simulink library "Audiopilot_3_5"  (R2022b)
settings: Solver=VariableStepAuto  StartTime=0.0  StopTime=10.0  RelTol=1e-3
values from neighbouring files (symbols this model uses):
  NumHFRefLPF = 4    [Audiopilot_3_5Mask.m]
  NumLFRef = 1    [Audiopilot_3_5Mask.m]
  NumMicChannels = 1    [Audiopilot_3_5Mask.m]
  NumMusicChannels = 6    [Audiopilot_3_5Mask.m]
undefined symbols (not defined in the file or in its folder): Row
libraries: TuneVar x11, StateVar x5, HandyTextFile x4, RTC x4, TOP x4, FeaturePath x3, Compensation x2, HighFrequencyNoiseEstimatorCoh x2, SpeedBoundsNoiseSlew x2, LowFrequencyNoiseEstimatorCoh x1
settings Model: Creator=sc10652  LastModifiedBy=db1045444
settings SolverCC: AlgebraicLoopSolver=TrustRegion
settings DataIOCC: ReturnWorkspaceOutputs=off
settings DebuggingCC: UnconnectedInputMsg=warning  UnconnectedOutputMsg=warning  UnconnectedLineMsg=warning  SFMachineParentedDataDiag=warning  ArithmeticOperatorsInVariantConditions=warning
settings ModelReferenceCC: EnableRefExpFcnMdlSchedulingChecks=on
settings SFSimCC: CustomCodeUndefinedFunction=UseInterfaceOnly

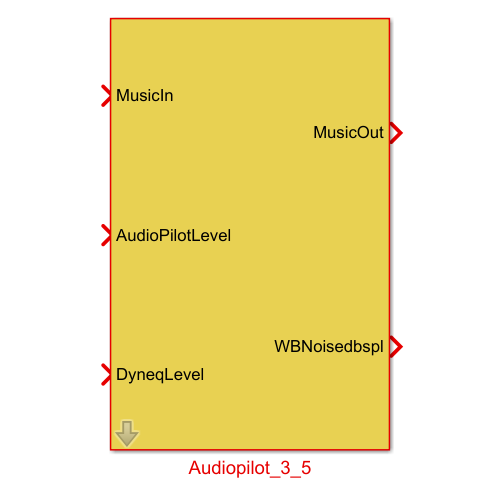
[thumbnail: Simulink's stored preview of the top-level diagram]
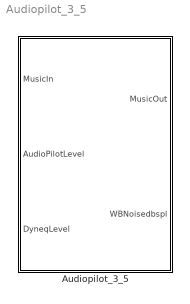
== system Audiopilot_3_5 ==
  Audiopilot_3_5 : Subsystem  mask(AudioPilot 3.5){FeatureName=Audiopilot, InputAudioMode=Stereo - 2 Channels, NoiseEstimationMode=Speed Only, IncludeSpumTails=on, IncludeIgnoreMicFlag=on, Config=[]}
      mask prompts: FeatureName "Feature Name:"; InputAudioMode "Input Audio Mode"; NoiseEstimationMode "Mode"; IncludeSpumTails "Include SPUM Tails as Reference Channels for High-Frequency Noise Estimator"; IncludeIgnoreMicFlag "Include Ignore Microphone Flag as Input"; Config "Audiopilot_3_5Config"
      mask help:
      | This is the top level model implementing AudioPilot 3.5.
      | It is configurable to accommodate both stereo inputs and surround inputs.  It can also reconfigure itself to become a speed-only implementation. For the regular implementation, there are two options. One is to allow a flag signal to instruct the algorithm to ignore the microphone signal; the other is to include in the set of "high-passed" reference channels the 2 channels representing the SPUM tails from the Medusa Upmixer.
      | Build Time Configuration settings typically set for this block include the frame size and the sample rate of the input audio. Other options include the type of code generation and whether all RTC blocks will generate a response.
      mask init:
      | blkh = gcbh;
      | 
      | Config = BTConfig.Assert(blkh,Config);
      | Config.Validate();
      | 
      | FrameSize = Config.FrameSize;
      | SampleRate = Config.SampleRateHz;
      |  
      | % Make the choice for the Noise Estimation Variant
      | Audiopilot_3_5Mask.ConfigureVariant(blkh,NoiseEstimationMode);
      | 
      | % Set up the number of audio channels for each input
      | [NumMicChannels,NumMusicChannels, ...
      |     NumHFRefLPF,NumHFRefBPF,NumLFRef] = ...
      |     Audiopilot_3_5Mask.ChannelSetUp(blkh,InputAudioMode,...
      |                 NoiseEstimationMode,IncludeSpumTails);
      | 
      | % Configure RTC responses            
      | Audiopilot_3_5Mask.ConfigureRtcResponses(blkh,...
      |                 Config.EnableRtcResponse)           
      | 
      | % Configure the Model according to Mask Parameters   
      | Audiopilot_3_5Mask.ConfigureModel(blkh,InputAudioMode,...
      |     NoiseEstimationMode,IncludeIgnoreMicFlag);
      | 
      | BTConfig.InitSetFeatureIfPresent(blkh,'FeatureName');
      mask TypeOptions FeatureName: FeaturePath/FeatureName
      mask TypeOptions InputAudioMode: Stereo - 2 Channels | Surround - 6 Channels
      mask TypeOptions NoiseEstimationMode: Regular | Speed Only
      mask Callback NoiseEstimationMode: Audiopilot_3_5Mask.NoiseEstimationModeCallBack(gcbh);
      mask Callback Config: BTConfig.CallbackHideIfPresent(gcbh,{'FeatureName'});
      mask DialogControl DTCTitle Prompt: <b> Design Time Configuration </b>
      mask DialogControl NoiseEstimationBox Prompt: Noise Estimation
      mask DialogControl BTCTitle Prompt: <b> Build Time Configuration </b>

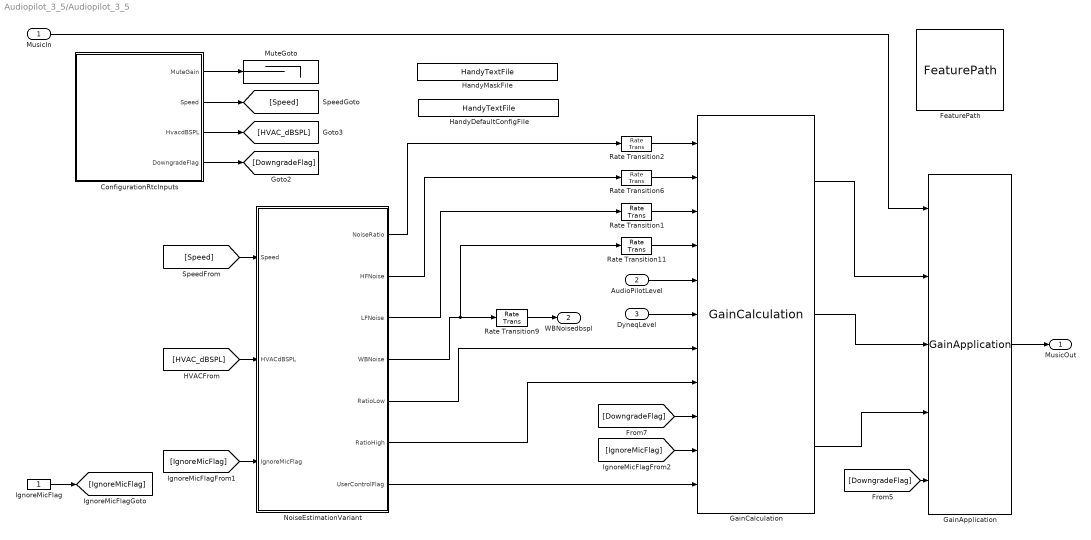
== system Audiopilot_3_5/Audiopilot_3_5 ==
  MusicIn : Inport  OutDataTypeStr=single  PortDimensions=[FrameSize NumMusicChannels]
  AudioPilotLevel : Inport  Port=2  OutDataTypeStr=single  PortDimensions=1
  DyneqLevel : Inport  Port=3  OutDataTypeStr=single  PortDimensions=1
  ConfigurationRtcInputs : Subsystem
  FeaturePath : FeaturePath/FeaturePath  FeatureName=Audiopilot  IsGroup=off  GroupNumber=-1  IsModule=off  TriggerInit=[1175 264 1290 371]
      settings: SourceProductName=Bose Talaria
  GainApplication : Compensation/GainApplication  NumInputChannels=NumMusicChannels  Config=Config.GainApp
  GainCalculation : Compensation/GainCalculation  Config=Config.GainCalc
  HandyDefaultConfigFile : HandyTextFile/HandyTextFile  TemplateSource=Config  FileSuffix=Init  OpenDialogOnLoad=off  UseThisBlockName=off  TheDefaultText=|  ShowInLibBrowser=on
      | % $(FILENAME) Setup model parameters for each "Init" callback (e.g. update diagram)
      | sample_rate_in_hertz = 44100;
      | frame_size = 32;
      | sysin_channel_count = 2;
      settings: SourceProductName=Bose Talaria
  HandyMaskFile : HandyTextFile/HandyTextFile  TemplateSource=Mask  FileSuffix=Init  OpenDialogOnLoad=off  UseThisBlockName=off  TheDefaultText=|  ShowInLibBrowser=on
      | % $(FILENAME) Setup model parameters for each "Init" callback (e.g. update diagram)
      | sample_rate_in_hertz = 44100;
      | frame_size = 32;
      | sysin_channel_count = 2;
      settings: SourceProductName=Bose Talaria
  IgnoreMicFlag : Constant  OutDataTypeStr=boolean
  MuteGoto : Terminator
  NoiseEstimationVariant : Subsystem  Variant=on  VariantControlMode=label  LabelModeActiveChoice=Speed Only  PropagateVariantConditions=on
  Rate Transition{1..2,6,9,11} (5 alike) : RateTransition  Deterministic=off
  MusicOut : Outport  VectorParamsAs1DForOutWhenUnconnected=off
  WBNoisedbspl : Outport  Port=2  VectorParamsAs1DForOutWhenUnconnected=off
  wires:
  [HVAC_dBSPL] -> NoiseEstimationVariant/2(HVACdBSPL)
  [Speed] -> NoiseEstimationVariant/1(Speed)
  NoiseEstimationVariant/3(LFNoise) -> Rate Transition1/1
  NoiseEstimationVariant/2(HFNoise) -> Rate Transition6/1
  NoiseEstimationVariant/1(NoiseRatio) -> Rate Transition2/1
  ConfigurationRtcInputs/1(MuteGain) -> MuteGoto/1
  ConfigurationRtcInputs/3(HvacdBSPL) -> [HVAC_dBSPL]
  ConfigurationRtcInputs/2(Speed) -> [Speed]
  ConfigurationRtcInputs/4(DowngradeFlag) -> [DowngradeFlag]
  [DowngradeFlag] -> GainCalculation/9
  GainCalculation/2 -> GainApplication/3
  NoiseEstimationVariant/4(WBNoise) -> Rate Transition11/1, Rate Transition9/1
  Rate Transition6/1 -> GainCalculation/2
  MusicIn/1 -> GainApplication/1
  NoiseEstimationVariant/7("UserControlFlag ") -> GainCalculation/11
  Rate Transition1/1 -> GainCalculation/3
  Rate Transition11/1 -> GainCalculation/4
  GainCalculation/1 -> GainApplication/2
  [DowngradeFlag] -> GainApplication/5
  DyneqLevel/1 -> GainCalculation/6
  Rate Transition2/1 -> GainCalculation/1
  AudioPilotLevel/1 -> GainCalculation/5
  GainApplication/1 -> MusicOut/1
  GainCalculation/3 -> GainApplication/4
  Rate Transition9/1 -> WBNoisedbspl/1
  NoiseEstimationVariant/5(RatioLow) -> GainCalculation/7
  NoiseEstimationVariant/6(RatioHigh) -> GainCalculation/8
  [IgnoreMicFlag] -> GainCalculation/10
  IgnoreMicFlag/1 -> [IgnoreMicFlag]
  [IgnoreMicFlag] -> NoiseEstimationVariant/3(IgnoreMicFlag)

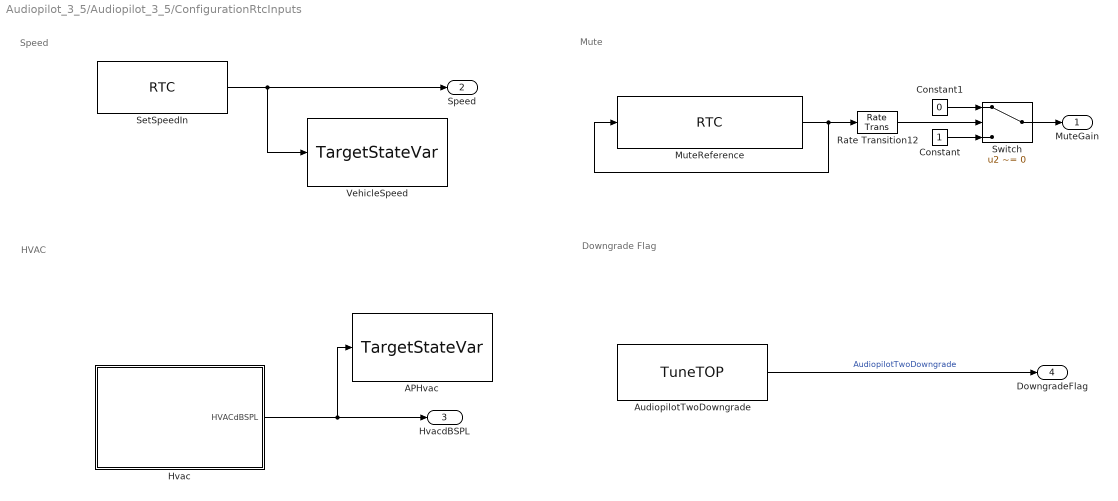
== system Audiopilot_3_5/Audiopilot_3_5/ConfigurationRtcInputs ==
  note: Mute
  note: Speed
  note: HVAC
  note: Downgrade Flag
  APHvac : StateVar/TargetStateVar  TriggerInit=[1390 1281 1530 1349]  TspName=HvacDbspl  StateName=HvacDbspl  UseSameName=on  IfdefMacro=[]
      settings: SourceProductName=Bose Talaria
  AudiopilotTwoDowngrade : TuneVar/TuneTOP  TriggerInit=[1655 1312 1805 1368]  TopName=TwoDowngrade  TuneName=TwoDowngrade  DataType=uint32  TunabilityNumber=1  MinValue=[]  MaxValue=[]  BankNumber=0  PreOverlay=false  PostOverlay=false  UseSameName=on  MaskValue=0
      settings: SourceProductName=Bose Talaria
  Constant : Constant  OutDataTypeStr=single
  Constant1 : Constant  Value=0  OutDataTypeStr=single
  Hvac : Subsystem  mask(AudioPilot - HVAC Table){Config=Config.HVAC}
      mask prompts: Config "HVACConfig"
      mask help: This block implements the table lookup for the HVAC index. It has 16 entries and returns the HVAC level in dBSPL.
      mask init:
      | blkh = gcbh;
      | 
      | Config = BTConfig.Assert(blkh,Config);
      | Config.Validate();
      | 
      | MaskHvacTableSize = Config.HVACTableSize;
      mask Help:
      | This block implements the table lookup for the HVAC index.  It has 16 entries and returns the HVAC level in dBSPL.
      | 
      | Arguments for this block:
      | 
      | Configuration
      | The block can be configured using an object of class, HVACConfig.  If the "use Default Configuration Only" box is checked, then this option is disabled.
      mask DialogControl BTC Prompt: Build Time Configuration
      mask DialogControl Config Tooltip: The configuration has to be an object of the class, HVACConfig.
  MuteReference : RTC/RTC  REQ_Priority=RTC_Mask.NormalPriority  RequestAtInit=off  EnableRequest=off  REQElemName1=muteReference  REQElemType1=uint32  REQElemWidth1=1  REQElemInitial1=0  REQElemType2=uint32  REQElemWidth2=1  REQElemInitial2=[]  REQElemType3=uint32  REQElemWidth3=1  REQElemInitial3=[]  REQElemType4=uint32  REQElemWidth4=1  REQElemInitial4=[]  REQElemType5=uint32  REQElemWidth5=1  REQElemInitial5=[]  REQElemType6=uint32  REQElemWidth6=1  REQElemInitial6=[]  REQElemType7=uint32  REQElemWidth7=1  REQElemInitial7=[]  REQElemType8=uint32  REQElemWidth8=1  REQElemInitial8=[]  REQElemType9=uint32  REQElemWidth9=1  REQElemInitial9=[]  REQElemType10=uint32  REQElemWidth10=1  REQElemInitial10=[]  EnableResponse=on  EnableRSP_StatusIn=off  RSPElemName1=muteReference  RSPElemType1=uint32  RSPElemWidth1=1  RSPElemType2=uint32  RSPElemWidth2=1  RSPElemType3=uint32  RSPElemWidth3=1  RSPElemType4=uint32  RSPElemWidth4=1  RSPElemType5=uint32  RSPElemWidth5=1  RSPElemType6=uint32  RSPElemWidth6=1  RSPElemType7=uint32  RSPElemWidth7=1  RSPElemType8=uint32  RSPElemWidth8=1  RSPElemType9=uint32  RSPElemWidth9=1  RSPElemType10=uint32  RSPElemWidth10=1  EnableNotification=off  EnableNTF_PrepTrig=off  NTFElemName1=freezeAdapt  NTFElemType1=single  NTFElemWidth1=1  NTFElemType2=uint32  NTFElemWidth2=1  NTFElemType3=uint32  NTFElemWidth3=1  NTFElemType4=uint32  NTFElemWidth4=1  NTFElemType5=uint32  NTFElemWidth5=1  NTFElemType6=uint32  NTFElemWidth6=1  NTFElemType7=uint32  NTFElemWidth7=1  NTFElemType8=uint32  NTFElemWidth8=1  NTFElemType9=uint32  NTFElemWidth9=1  NTFElemType10=uint32  NTFElemWidth10=1  MaskMessageName=muteReference
      settings: SourceProductName=Bose Talaria
  Rate Transition12 : RateTransition  Deterministic=off
  SetSpeedIn : RTC/RTC  REQ_Priority=RTC_Mask.NormalPriority  RequestAtInit=off  EnableRequest=off  REQElemName1=speedIn  REQElemType1=single  REQElemWidth1=1  REQElemInitial1=[]  REQElemType2=single  REQElemWidth2=1  REQElemInitial2=[]  REQElemType3=uint32  REQElemWidth3=1  REQElemInitial3=[]  REQElemType4=uint32  REQElemWidth4=1  REQElemInitial4=[]  REQElemType5=uint32  REQElemWidth5=1  REQElemInitial5=[]  REQElemType6=uint32  REQElemWidth6=1  REQElemInitial6=[]  REQElemType7=uint32  REQElemWidth7=1  REQElemInitial7=[]  REQElemType8=uint32  REQElemWidth8=1  REQElemInitial8=[]  REQElemType9=uint32  REQElemWidth9=1  REQElemInitial9=[]  REQElemType10=uint32  REQElemWidth10=1  REQElemInitial10=[]  EnableResponse=off  EnableRSP_StatusIn=off  RSPElemType1=single  RSPElemWidth1=1  RSPElemType2=uint32  RSPElemWidth2=1  RSPElemType3=uint32  RSPElemWidth3=1  RSPElemType4=uint32  RSPElemWidth4=1  RSPElemType5=uint32  RSPElemWidth5=1  RSPElemType6=uint32  RSPElemWidth6=1  RSPElemType7=uint32  RSPElemWidth7=1  RSPElemType8=uint32  RSPElemWidth8=1  RSPElemType9=uint32  RSPElemWidth9=1  RSPElemType10=uint32  RSPElemWidth10=1  EnableNotification=off  EnableNTF_PrepTrig=off  NTFElemType1=uint32  NTFElemWidth1=1  NTFElemType2=uint32  NTFElemWidth2=1  NTFElemType3=uint32  NTFElemWidth3=1  NTFElemType4=uint32  NTFElemWidth4=1  NTFElemType5=uint32  NTFElemWidth5=1  NTFElemType6=uint32  NTFElemWidth6=1  NTFElemType7=uint32  NTFElemWidth7=1  NTFElemType8=uint32  NTFElemWidth8=1  NTFElemType9=uint32  NTFElemWidth9=1  NTFElemType10=uint32  NTFElemWidth10=1  MaskMessageName=setSpeedIn
      settings: SourceProductName=Bose Talaria
  Switch : Switch  Criteria=u2 ~= 0  OutDataTypeStr=single  SaturateOnIntegerOverflow=off  InputSameDT=off
  VehicleSpeed : StateVar/TargetStateVar  TriggerInit=[1345 1086 1485 1154]  TspName=VehicleSpeed  StateName=VehicleSpeed  UseSameName=on  IfdefMacro=[]
      settings: SourceProductName=Bose Talaria
  MuteGain : Outport  OutDataTypeStr=single  VectorParamsAs1DForOutWhenUnconnected=off
  Speed : Outport  Port=2  VectorParamsAs1DForOutWhenUnconnected=off
  HvacdBSPL : Outport  Port=3  VectorParamsAs1DForOutWhenUnconnected=off
  DowngradeFlag : Outport  Port=4  VectorParamsAs1DForOutWhenUnconnected=off
  wires:
  MuteReference/1 -> Rate Transition12/1, MuteReference/1
  Rate Transition12/1 -> Switch/2
  SetSpeedIn/1 -> VehicleSpeed/1, Speed/1
  AudiopilotTwoDowngrade/1 -> DowngradeFlag/1  "AudiopilotTwoDowngrade"
  Hvac/1(HVACdBSPL) -> APHvac/1, HvacdBSPL/1
  Constant/1 -> Switch/3
  Switch/1 -> MuteGain/1
  Constant1/1 -> Switch/1

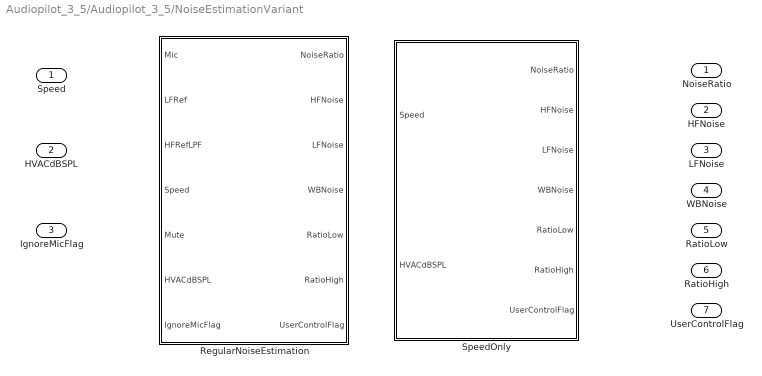
== system Audiopilot_3_5/Audiopilot_3_5/NoiseEstimationVariant ==
  Speed : Inport
  HVACdBSPL : Inport  Port=2
  IgnoreMicFlag : Inport  Port=3
  RegularNoiseEstimation : Subsystem  VariantControl=Regular
  SpeedOnly : Subsystem  VariantControl=Speed Only  mask(AudioPilot - Speed Only Noise Estimation){Config=Config.SpeedOnly}
      mask prompts: Config "SpeedOnlyConfig"
      mask help: This block implements the speed only variant for noise estimation
      mask init:
      | blkh = gcbh;
      | 
      | Config = BTConfig.Assert(blkh,Config);
      | Config.Validate();
      | 
      | SampleRate = Config.SampleRateHz;
      | DecRate = Config.DecRateHz;
      mask Help:
      | This block implements the speed only variant for noise estimation.
      | 
      | Arguments for this block:
      | 
      | Configuration
      | The block can be configured using an object of class, SpeedOnlyConfig.  If the "use Default Configuration Only" box is checked, then this option is disabled.
      | 
      | Sample Rate
      | This is the sample rate of the input audio streams, typically 44100 Hz or 48 kHz.
      mask DialogControl BTC Prompt: Build Time Configuration
      mask DialogControl Config Tooltip: The configuration has to be an object of the class, SpeedOnlyConfig.
  NoiseRatio : Outport  VectorParamsAs1DForOutWhenUnconnected=off
  HFNoise : Outport  Port=2  VectorParamsAs1DForOutWhenUnconnected=off
  LFNoise : Outport  Port=3  VectorParamsAs1DForOutWhenUnconnected=off
  WBNoise : Outport  Port=4  VectorParamsAs1DForOutWhenUnconnected=off
  RatioLow : Outport  Port=5  VectorParamsAs1DForOutWhenUnconnected=off
  RatioHigh : Outport  Port=6  VectorParamsAs1DForOutWhenUnconnected=off
  "UserControlFlag " : Outport  Port=7  VectorParamsAs1DForOutWhenUnconnected=off

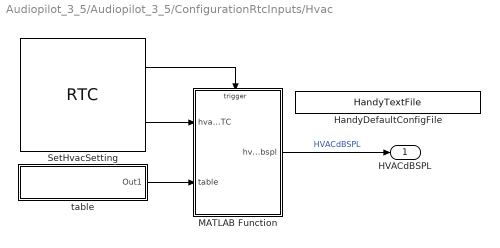
== system Audiopilot_3_5/Audiopilot_3_5/ConfigurationRtcInputs/Hvac ==
  HandyDefaultConfigFile : HandyTextFile/HandyTextFile  TemplateSource=Config  FileSuffix=Init  OpenDialogOnLoad=off  UseThisBlockName=off  TheDefaultText=|  ShowInLibBrowser=on
      | % $(FILENAME) Setup model parameters for each "Init" callback (e.g. update diagram)
      | sample_rate_in_hertz = 44100;
      | frame_size = 32;
      | sysin_channel_count = 2;
      settings: SourceProductName=Bose Talaria
  MATLAB Function : MATLAB Function  TreatAsAtomicUnit=on
  SetHvacSetting : RTC/RTC  REQ_Priority=RTC_Mask.NormalPriority  RequestAtInit=off  EnableRequest=on  REQElemName1=HVACSetting  REQElemType1=single  REQElemWidth1=1  REQElemInitial1=[]  REQElemType2=single  REQElemWidth2=1  REQElemInitial2=[]  REQElemType3=uint32  REQElemWidth3=1  REQElemInitial3=[]  REQElemType4=uint32  REQElemWidth4=1  REQElemInitial4=[]  REQElemType5=uint32  REQElemWidth5=1  REQElemInitial5=[]  REQElemType6=uint32  REQElemWidth6=1  REQElemInitial6=[]  REQElemType7=uint32  REQElemWidth7=1  REQElemInitial7=[]  REQElemType8=uint32  REQElemWidth8=1  REQElemInitial8=[]  REQElemType9=uint32  REQElemWidth9=1  REQElemInitial9=[]  REQElemType10=uint32  REQElemWidth10=1  REQElemInitial10=[]  EnableResponse=off  EnableRSP_StatusIn=off  RSPElemType1=uint32  RSPElemWidth1=1  RSPElemType2=uint32  RSPElemWidth2=1  RSPElemType3=uint32  RSPElemWidth3=1  RSPElemType4=uint32  RSPElemWidth4=1  RSPElemType5=uint32  RSPElemWidth5=1  RSPElemType6=uint32  RSPElemWidth6=1  RSPElemType7=uint32  RSPElemWidth7=1  RSPElemType8=uint32  RSPElemWidth8=1  RSPElemType9=uint32  RSPElemWidth9=1  RSPElemType10=uint32  RSPElemWidth10=1  EnableNotification=off  EnableNTF_PrepTrig=off  NTFElemType1=uint32  NTFElemWidth1=1  NTFElemType2=uint32  NTFElemWidth2=1  NTFElemType3=uint32  NTFElemWidth3=1  NTFElemType4=uint32  NTFElemWidth4=1  NTFElemType5=uint32  NTFElemWidth5=1  NTFElemType6=uint32  NTFElemWidth6=1  NTFElemType7=uint32  NTFElemWidth7=1  NTFElemType8=uint32  NTFElemWidth8=1  NTFElemType9=uint32  NTFElemWidth9=1  NTFElemType10=uint32  NTFElemWidth10=1  MaskMessageName=setHVACSetting
      settings: SourceProductName=Bose Talaria
  table : Subsystem
  HVACdBSPL : Outport  VectorParamsAs1DForOutWhenUnconnected=off
  wires:
  SetHvacSetting/2 -> MATLAB Function/1(hvacSettingRTC)
  SetHvacSetting/1 -> MATLAB Function/Trigger
  table/1(Out1) -> MATLAB Function/2(table)
  MATLAB Function/1(hvacDbspl) -> HVACdBSPL/1  "HVACdBSPL"

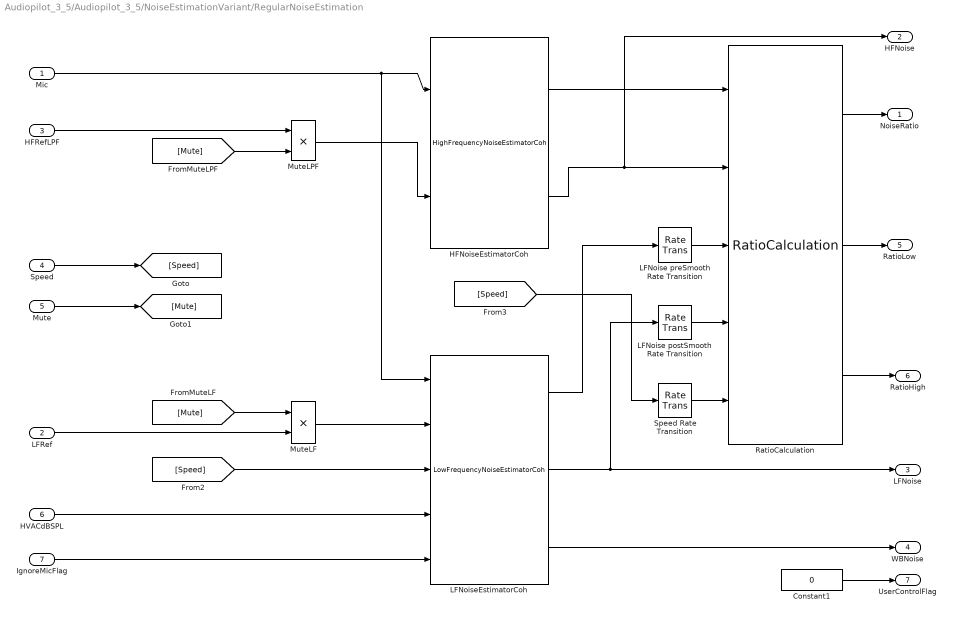
== system Audiopilot_3_5/Audiopilot_3_5/NoiseEstimationVariant/RegularNoiseEstimation ==
  Mic : Inport  PortDimensions=[FrameSize NumMicChannels]
  LFRef : Inport  Port=2  OutDataTypeStr=single  PortDimensions=[FrameSize NumLFRef]
  HFRefLPF : Inport  Port=3  OutDataTypeStr=single  PortDimensions=[FrameSize NumHFRefLPF]
  Speed : Inport  Port=4  OutDataTypeStr=single
  Mute : Inport  Port=5  OutDataTypeStr=single
  HVACdBSPL : Inport  Port=6  OutDataTypeStr=single
  IgnoreMicFlag : Inport  Port=7
  Constant1 : Constant  Value=0  OutDataTypeStr=boolean
  HFNoiseEstimatorCoh : HighFrequencyNoiseEstimatorCoh/HighFrequencyNoiseEstimatorCoh  FeatureName=HfNoise  NumHFRefLPF=NumHFRefLPF  NumHFRefBPF=NumHFRefBPF  Config=Config.HfNoise  TriggerInit=0
  LFNoise postSmooth Rate Transition : RateTransition  Deterministic=off
  LFNoise preSmooth Rate Transition : RateTransition  Deterministic=off
  LFNoiseEstimatorCoh : LowFrequencyNoiseEstimatorCoh/LowFrequencyNoiseEstimatorCoh  FeatureName=LfNoise  Config=Config.LfNoise  TriggerInit=0
  MuteLF : Product  Inputs=**
  MuteLPF : Product  Inputs=**
  RatioCalculation : HighFrequencyNoiseEstimatorCoh/RatioCalculation  FeatureName=Ratio  Config=Config.Ratio
  Speed Rate Transition : RateTransition  Deterministic=off
  NoiseRatio : Outport  VectorParamsAs1DForOutWhenUnconnected=off
  HFNoise : Outport  Port=2  VectorParamsAs1DForOutWhenUnconnected=off
  LFNoise : Outport  Port=3  VectorParamsAs1DForOutWhenUnconnected=off
  WBNoise : Outport  Port=4  VectorParamsAs1DForOutWhenUnconnected=off
  RatioLow : Outport  Port=5  VectorParamsAs1DForOutWhenUnconnected=off
  RatioHigh : Outport  Port=6  VectorParamsAs1DForOutWhenUnconnected=off
  UserControlFlag : Outport  Port=7  VectorParamsAs1DForOutWhenUnconnected=off
  wires:
  Speed/1 -> [Speed]
  Mute/1 -> [Mute]
  Constant1/1 -> UserControlFlag/1
  RatioCalculation/1 -> NoiseRatio/1
  LFNoiseEstimatorCoh/3 -> WBNoise/1
  [Mute] -> MuteLF/1
  HFNoiseEstimatorCoh/1 -> RatioCalculation/1
  MuteLF/1 -> LFNoiseEstimatorCoh/2
  [Speed] -> LFNoiseEstimatorCoh/3
  LFNoiseEstimatorCoh/1 -> LFNoise preSmooth Rate Transition/1
  [Speed] -> Speed Rate Transition/1
  HFRefLPF/1 -> MuteLPF/1
  MuteLPF/1 -> HFNoiseEstimatorCoh/2
  [Mute] -> MuteLPF/2
  Mic/1 -> LFNoiseEstimatorCoh/1, HFNoiseEstimatorCoh/1
  HFNoiseEstimatorCoh/2 -> HFNoise/1, RatioCalculation/2
  HVACdBSPL/1 -> LFNoiseEstimatorCoh/4
  LFNoiseEstimatorCoh/2 -> LFNoise postSmooth Rate Transition/1, LFNoise/1
  LFRef/1 -> MuteLF/2
  LFNoise preSmooth Rate Transition/1 -> RatioCalculation/3
  LFNoise postSmooth Rate Transition/1 -> RatioCalculation/4
  Speed Rate Transition/1 -> RatioCalculation/5
  RatioCalculation/2 -> RatioLow/1
  RatioCalculation/3 -> RatioHigh/1
  IgnoreMicFlag/1 -> LFNoiseEstimatorCoh/5

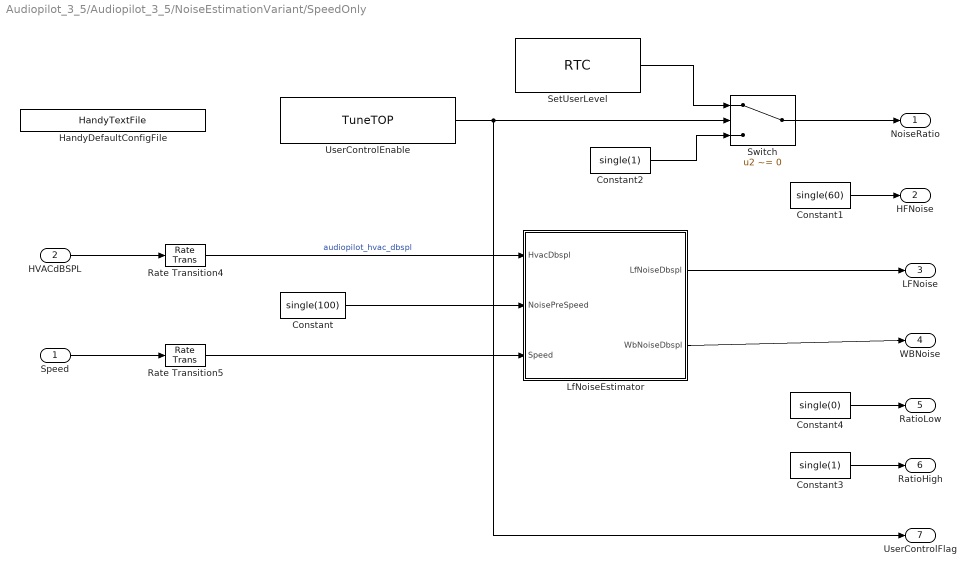
== system Audiopilot_3_5/Audiopilot_3_5/NoiseEstimationVariant/SpeedOnly ==
  Speed : Inport  OutDataTypeStr=single
  HVACdBSPL : Inport  Port=2  OutDataTypeStr=single
  Constant : Constant  Value=single(100)  OutDataTypeStr=single
  Constant1 : Constant  Value=single(60)  OutDataTypeStr=single
  Constant2 : Constant  Value=single(1)  OutDataTypeStr=single
  Constant3 : Constant  Value=single(1)  OutDataTypeStr=single
  Constant4 : Constant  Value=single(0)  OutDataTypeStr=single
  HandyDefaultConfigFile : HandyTextFile/HandyTextFile  TemplateSource=Config  FileSuffix=Init  OpenDialogOnLoad=off  UseThisBlockName=off  TheDefaultText=|  ShowInLibBrowser=on
      | % $(FILENAME) Setup model parameters for each "Init" callback (e.g. update diagram)
      | sample_rate_in_hertz = 44100;
      | frame_size = 32;
      | sysin_channel_count = 2;
      settings: SourceProductName=Bose Talaria
  LfNoiseEstimator : Subsystem
  Rate Transition4 : RateTransition  Deterministic=off  OutPortSampleTime=1/DecRate
  Rate Transition5 : RateTransition  Deterministic=off  OutPortSampleTime=1/DecRate
  SetUserLevel : RTC/RTC  REQ_Priority=RTC_Mask.NormalPriority  RequestAtInit=off  EnableRequest=off  REQElemName1=userLevel  REQElemType1=single  REQElemWidth1=1  REQElemInitial1=[]  REQElemType2=single  REQElemWidth2=1  REQElemInitial2=[]  REQElemType3=uint32  REQElemWidth3=1  REQElemInitial3=[]  REQElemType4=uint32  REQElemWidth4=1  REQElemInitial4=[]  REQElemType5=uint32  REQElemWidth5=1  REQElemInitial5=[]  REQElemType6=uint32  REQElemWidth6=1  REQElemInitial6=[]  REQElemType7=uint32  REQElemWidth7=1  REQElemInitial7=[]  REQElemType8=uint32  REQElemWidth8=1  REQElemInitial8=[]  REQElemType9=uint32  REQElemWidth9=1  REQElemInitial9=[]  REQElemType10=uint32  REQElemWidth10=1  REQElemInitial10=[]  EnableResponse=off  EnableRSP_StatusIn=off  RSPElemName1=FANLevel  RSPElemType1=single  RSPElemWidth1=1  RSPElemType2=uint32  RSPElemWidth2=1  RSPElemType3=uint32  RSPElemWidth3=1  RSPElemType4=uint32  RSPElemWidth4=1  RSPElemType5=uint32  RSPElemWidth5=1  RSPElemType6=uint32  RSPElemWidth6=1  RSPElemType7=uint32  RSPElemWidth7=1  RSPElemType8=uint32  RSPElemWidth8=1  RSPElemType9=uint32  RSPElemWidth9=1  RSPElemType10=uint32  RSPElemWidth10=1  EnableNotification=off  EnableNTF_PrepTrig=off  NTFElemType1=uint32  NTFElemWidth1=1  NTFElemType2=uint32  NTFElemWidth2=1  NTFElemType3=uint32  NTFElemWidth3=1  NTFElemType4=uint32  NTFElemWidth4=1  NTFElemType5=uint32  NTFElemWidth5=1  NTFElemType6=uint32  NTFElemWidth6=1  NTFElemType7=uint32  NTFElemWidth7=1  NTFElemType8=uint32  NTFElemWidth8=1  NTFElemType9=uint32  NTFElemWidth9=1  NTFElemType10=uint32  NTFElemWidth10=1  MaskMessageName=setUserLevel
      settings: SourceProductName=Bose Talaria
  Switch : Switch  Criteria=u2 ~= 0  Threshold=0.5  SaturateOnIntegerOverflow=off  InputSameDT=off
  UserControlEnable : TuneVar/TuneTOP  TriggerInit=[480 112 655 158]  TopName=UserControlEnable  TuneName=UserControlEnable  DataType=single  TunabilityNumber=1  MinValue=[]  MaxValue=[]  BankNumber=0  PreOverlay=false  PostOverlay=false  UseSameName=on  MaskValue=1
      settings: SourceProductName=Bose Talaria
  NoiseRatio : Outport  VectorParamsAs1DForOutWhenUnconnected=off
  HFNoise : Outport  Port=2  VectorParamsAs1DForOutWhenUnconnected=off
  LFNoise : Outport  Port=3  VectorParamsAs1DForOutWhenUnconnected=off
  WBNoise : Outport  Port=4  VectorParamsAs1DForOutWhenUnconnected=off
  RatioLow : Outport  Port=5  VectorParamsAs1DForOutWhenUnconnected=off
  RatioHigh : Outport  Port=6  VectorParamsAs1DForOutWhenUnconnected=off
  UserControlFlag : Outport  Port=7  VectorParamsAs1DForOutWhenUnconnected=off
  wires:
  Constant4/1 -> RatioLow/1
  Constant3/1 -> RatioHigh/1
  Constant1/1 -> HFNoise/1
  Switch/1 -> NoiseRatio/1
  Constant2/1 -> Switch/3
  UserControlEnable/1 -> Switch/2, UserControlFlag/1
  SetUserLevel/1 -> Switch/1
  HVACdBSPL/1 -> Rate Transition4/1
  Speed/1 -> Rate Transition5/1
  Rate Transition4/1 -> LfNoiseEstimator/1(HvacDbspl)  "audiopilot_hvac_dbspl"
  Constant/1 -> LfNoiseEstimator/2(NoisePreSpeed)
  Rate Transition5/1 -> LfNoiseEstimator/3(Speed)
  LfNoiseEstimator/1(LfNoiseDbspl) -> LFNoise/1
  LfNoiseEstimator/2(WbNoiseDbspl) -> WBNoise/1

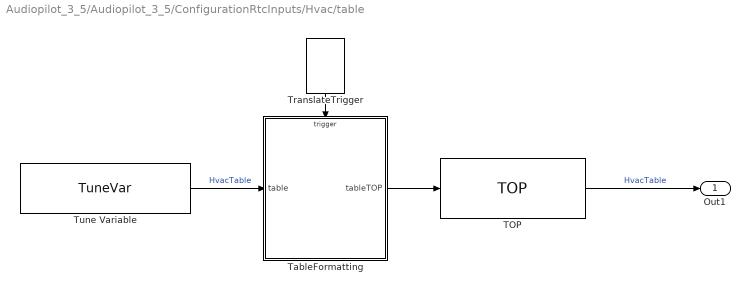
== system Audiopilot_3_5/Audiopilot_3_5/ConfigurationRtcInputs/Hvac/table ==
  TOP : TOP/TOP  TriggerInit=[440 20 585 80]  TopName=HvacTable  DataType=single  BankNumber=0  PreOverlay=false  PostOverlay=false  Role=Automatic
      settings: SourceProductName=Bose Talaria
  TableFormatting : MATLAB Function  TreatAsAtomicUnit=on
  TranslateTrigger : TuneVar/TranslateTrigger  TriggerInit=[306 -100 344 -45]
      settings: SourceProductName=Bose Talaria
  Tune Variable : TuneVar/TuneVar  TuneName=HvacTable  SpecifyMaxSize=on  VariableDim=1 (Row)  MaxSize=[MaskHvacTableSize 2]  TunabilityNumber=1  MinValue=[]  MaxValue=[]  TriggerInit=[20 25 190 75]  MaskValue=Config.HVACTabledBSPL
      settings: SourceProductName=Bose Talaria
  Out1 : Outport  VectorParamsAs1DForOutWhenUnconnected=off
  wires:
  TOP/1 -> Out1/1  "HvacTable"
  Tune Variable/1 -> TableFormatting/1(table)  "HvacTable"
  TableFormatting/1(tableTOP) -> TOP/1
  TranslateTrigger/1 -> TableFormatting/Trigger

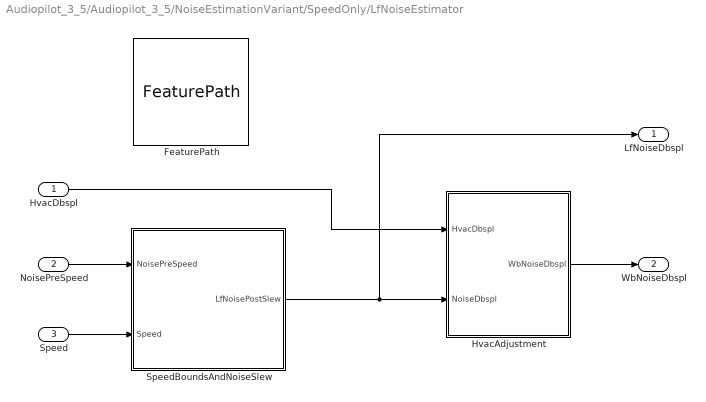
== system Audiopilot_3_5/Audiopilot_3_5/NoiseEstimationVariant/SpeedOnly/LfNoiseEstimator ==
  HvacDbspl : Inport
  NoisePreSpeed : Inport  Port=2
  Speed : Inport  Port=3
  FeaturePath : FeaturePath/FeaturePath  FeatureName=LfNoise  IsGroup=off  GroupNumber=-1  IsModule=off  TriggerInit=[255 -66 370 41]
      settings: SourceProductName=Bose Talaria
  "HvacAdjustment  " : Subsystem
  SpeedBoundsAndNoiseSlew : Subsystem
  LfNoiseDbspl : Outport  VectorParamsAs1DForOutWhenUnconnected=off
  WbNoiseDbspl : Outport  Port=2  VectorParamsAs1DForOutWhenUnconnected=off
  wires:
  SpeedBoundsAndNoiseSlew/1(LfNoisePostSlew) -> LfNoiseDbspl/1, "HvacAdjustment  "/2(NoiseDbspl)
  NoisePreSpeed/1 -> SpeedBoundsAndNoiseSlew/1(NoisePreSpeed)
  HvacDbspl/1 -> "HvacAdjustment  "/1(HvacDbspl)
  Speed/1 -> SpeedBoundsAndNoiseSlew/2(Speed)
  "HvacAdjustment  "/1(WbNoiseDbspl) -> WbNoiseDbspl/1

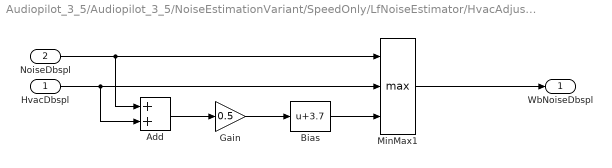
== system Audiopilot_3_5/Audiopilot_3_5/NoiseEstimationVariant/SpeedOnly/LfNoiseEstimator/HvacAdjustment   ==
  HvacDbspl : Inport
  NoiseDbspl : Inport  Port=2
  Add : Sum
  Bias : Bias  Bias=3.7  SaturateOnIntegerOverflow=off
  Gain : Gain  Gain=0.5
  MinMax1 : MinMax  Function=max  Inputs=3
  WbNoiseDbspl : Outport  VectorParamsAs1DForOutWhenUnconnected=off
  wires:
  NoiseDbspl/1 -> MinMax1/1, Add/1
  HvacDbspl/1 -> MinMax1/2, Add/2
  MinMax1/1 -> WbNoiseDbspl/1
  Add/1 -> Gain/1
  Gain/1 -> Bias/1
  Bias/1 -> MinMax1/3

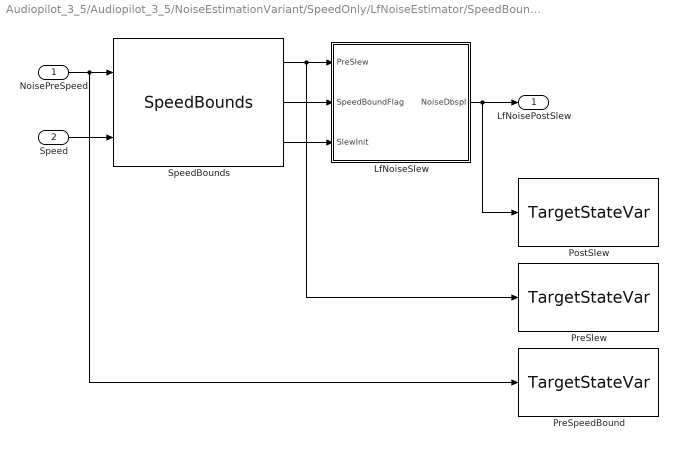
== system Audiopilot_3_5/Audiopilot_3_5/NoiseEstimationVariant/SpeedOnly/LfNoiseEstimator/SpeedBoundsAndNoiseSlew ==
  NoisePreSpeed : Inport
  Speed : Inport  Port=2
  LfNoiseSlew : Subsystem
  PostSlew : StateVar/TargetStateVar  TriggerInit=[1100 231 1240 299]  TspName=PostSlew  StateName=PostSlew  UseSameName=on  IfdefMacro=[]
      settings: SourceProductName=Bose Talaria
  PreSlew : StateVar/TargetStateVar  TriggerInit=[1100 316 1240 384]  TspName=PreSlew  StateName=PreSlew  UseSameName=on  IfdefMacro=[]
      settings: SourceProductName=Bose Talaria
  PreSpeedBound : StateVar/TargetStateVar  TriggerInit=[1100 401 1240 469]  TspName=PreSpeedBound  StateName=PreSpeedBound  UseSameName=on  IfdefMacro=[]
      settings: SourceProductName=Bose Talaria
  SpeedBounds : SpeedBoundsNoiseSlew/SpeedBounds  FeatureName=SpeedBounds  Config=Config.SpeedBounds
  LfNoisePostSlew : Outport  VectorParamsAs1DForOutWhenUnconnected=off
  wires:
  Speed/1 -> SpeedBounds/2
  SpeedBounds/2 -> LfNoiseSlew/2(SpeedBoundFlag)
  SpeedBounds/3 -> LfNoiseSlew/3(SlewInit)
  LfNoiseSlew/1(NoiseDbspl) -> PostSlew/1, LfNoisePostSlew/1
  NoisePreSpeed/1 -> PreSpeedBound/1, SpeedBounds/1
  SpeedBounds/1 -> PreSlew/1, LfNoiseSlew/1(PreSlew)

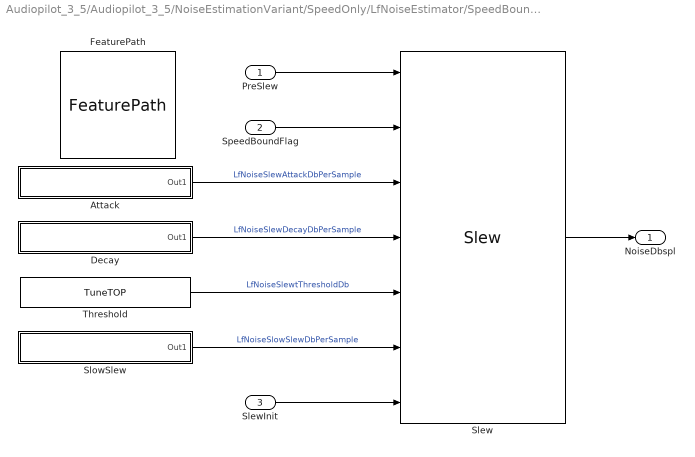
== system Audiopilot_3_5/Audiopilot_3_5/NoiseEstimationVariant/SpeedOnly/LfNoiseEstimator/SpeedBoundsAndNoiseSlew/LfNoiseSlew ==
  PreSlew : Inport
  SpeedBoundFlag : Inport  Port=2
  SlewInit : Inport  Port=3
  Attack : Subsystem
  Decay : Subsystem
  FeaturePath : FeaturePath/FeaturePath  FeatureName=Slew  IsGroup=off  GroupNumber=-1  IsModule=off  TriggerInit=[-225 64 -110 171]
      settings: SourceProductName=Bose Talaria
  Slew : SpeedBoundsNoiseSlew/Slew  SystemSampleTime=-1  VariantActivationTime=update diagram  Latency=0  AutoFrameSizeCalculation=off
  SlowSlew : Subsystem
  Threshold : TuneVar/TuneTOP  TriggerInit=[-265 290 -95 320]  TopName=ThresholdDb  TuneName=ThresholdDb  DataType=single  TunabilityNumber=1  MinValue=[]  MaxValue=[]  BankNumber=0  PreOverlay=false  PostOverlay=false  UseSameName=on  MaskValue=Config.SlewThresholdDb
      settings: SourceProductName=Bose Talaria
  NoiseDbspl : Outport  VectorParamsAs1DForOutWhenUnconnected=off
  wires:
  Slew/1 -> NoiseDbspl/1
  SpeedBoundFlag/1 -> Slew/2
  PreSlew/1 -> Slew/1
  SlowSlew/1(Out1) -> Slew/6  "LfNoiseSlowSlewDbPerSample"
  Attack/1(Out1) -> Slew/3  "LfNoiseSlewAttackDbPerSample"
  Threshold/1 -> Slew/5  "LfNoiseSlewtThresholdDb"
  Decay/1(Out1) -> Slew/4  "LfNoiseSlewDecayDbPerSample"
  SlewInit/1 -> Slew/7

== system Audiopilot_3_5/Audiopilot_3_5/NoiseEstimationVariant/SpeedOnly/LfNoiseEstimator/SpeedBoundsAndNoiseSlew/LfNoiseSlew/Attack ==
  TOP : TOP/TOP  TriggerInit=[125 85 270 145]  TopName=AttackDbPerSample  DataType=single  BankNumber=0  PreOverlay=false  PostOverlay=false  Role=Automatic
      settings: SourceProductName=Bose Talaria
  TranslateTrigger : TuneVar/TranslateTrigger  TriggerInit=[-19 -10 19 45]
      settings: SourceProductName=Bose Talaria
  Tune Variable : TuneVar/TuneVar  TuneName=AttackDbPerS  SpecifyMaxSize=off  VariableDim=1 (Row)  MaxSize=[1 1]  TunabilityNumber=1  MinValue=[]  MaxValue=[]  TriggerInit=[-325 90 -155 140]  MaskValue=Config.SlewAttackdDbpsec
      settings: SourceProductName=Bose Talaria
  sec2sample : MATLAB Function  TreatAsAtomicUnit=on
  Out1 : Outport  VectorParamsAs1DForOutWhenUnconnected=off
  wires:
  TOP/1 -> Out1/1  "AttackDbPerSample"
  sec2sample/1(y) -> TOP/1
  Tune Variable/1 -> sec2sample/1(u)  "AttackDbPerS"
  TranslateTrigger/1 -> sec2sample/Trigger

== system Audiopilot_3_5/Audiopilot_3_5/NoiseEstimationVariant/SpeedOnly/LfNoiseEstimator/SpeedBoundsAndNoiseSlew/LfNoiseSlew/Decay ==
  TOP : TOP/TOP  TriggerInit=[100 85 245 145]  TopName=DecayDbPerSample  DataType=single  BankNumber=0  PreOverlay=false  PostOverlay=false  Role=Automatic
      settings: SourceProductName=Bose Talaria
  TranslateTrigger : TuneVar/TranslateTrigger  TriggerInit=[-19 -10 19 45]
      settings: SourceProductName=Bose Talaria
  Tune Variable : TuneVar/TuneVar  TuneName=DecayDbPerS  SpecifyMaxSize=off  VariableDim=1 (Row)  MaxSize=[1 1]  TunabilityNumber=1  MinValue=[]  MaxValue=[]  TriggerInit=[-345 90 -175 140]  MaskValue=Config.SlewDecayDbpsec
      settings: SourceProductName=Bose Talaria
  sec2sample : MATLAB Function  TreatAsAtomicUnit=on
  Out1 : Outport  VectorParamsAs1DForOutWhenUnconnected=off
  wires:
  TranslateTrigger/1 -> sec2sample/Trigger
  Tune Variable/1 -> sec2sample/1(u)  "DecayDbPerS"
  sec2sample/1(y) -> TOP/1
  TOP/1 -> Out1/1  "DecayDbPerSample"

== system Audiopilot_3_5/Audiopilot_3_5/NoiseEstimationVariant/SpeedOnly/LfNoiseEstimator/SpeedBoundsAndNoiseSlew/LfNoiseSlew/SlowSlew ==
  TOP : TOP/TOP  TriggerInit=[100 85 245 145]  TopName=SlowDbPerSample  DataType=single  BankNumber=0  PreOverlay=false  PostOverlay=false  Role=Automatic
      settings: SourceProductName=Bose Talaria
  TranslateTrigger : TuneVar/TranslateTrigger  TriggerInit=[-19 -10 19 45]
      settings: SourceProductName=Bose Talaria
  Tune Variable : TuneVar/TuneVar  TuneName=SlowDbPerS  SpecifyMaxSize=off  VariableDim=1 (Row)  MaxSize=[1 1]  TunabilityNumber=1  MinValue=[]  MaxValue=[]  TriggerInit=[-330 90 -160 140]  MaskValue=Config.SlewSlowSlewDbpsec
      settings: SourceProductName=Bose Talaria
  sec2sample : MATLAB Function  TreatAsAtomicUnit=on
  Out1 : Outport  VectorParamsAs1DForOutWhenUnconnected=off
  wires:
  TOP/1 -> Out1/1  "SlowDbPerSample"
  sec2sample/1(y) -> TOP/1
  Tune Variable/1 -> sec2sample/1(u)  "SlowDbPerS"
  TranslateTrigger/1 -> sec2sample/Trigger

== matlab function Audiopilot_3_5/NoiseEstimationVariant/SpeedOnly/LfNoiseEstimator/SpeedBoundsAndNoiseSlew/LfNoiseSlew/Attack/sec2sample ==
  data: u input; y output; DecRate parameter
  events: trigger input FUNCTION_CALL_EVENT
function y = fcn(u, DecRate)
% Convert rate from per second to per sample

y = u.Value/DecRate;

== matlab function Audiopilot_3_5/ConfigurationRtcInputs/Hvac/MATLAB Function ==
  data: hvacSettingRTC input; hvacDbspl output; table input
  events: trigger input FUNCTION_CALL_EVENT
function hvacDbspl = fcn(hvacSettingRTC, table)

% "hvacSetting": Float value between [0,1.0], coming in as a control message
% "table": Table containing noise values corresponding to different
%          HVAC settings
% "hvacDbspl": Interpolated HVAC noise value (dBSPL)


% Ensuring the RTC hvac setting is always in the range [0,1.0]
if (hvacSettingRTC < 0.0)
    hvacSettingRTC = single(0.0);
elseif (hvacSettingRTC > 1.0)
    hvacSettingRTC = single(1.0);
end

% Since the HVACtable size is variable, the tune variable translation fills
% the empty elements with 0s. The tune translation ensures that the first
% HVAC setting will be a 0.0. Hence we extract the table upto the index of
% the trailing zero.
zeroIdx = find(table(:,1) == 0);
if length(zeroIdx) > 1
    trailingZeroIdx = zeroIdx(2);   
    tableSetting = table(1: trailingZeroIdx-1,1);
    tableNoise   = table(1: trailingZeroIdx-1,2);
else
    tableSetting = table(:,1);
    tableNoise   = table(:,2);
end
% [tableSetting, idx] = unique(table(:,1));
% tableNoise = table(idx,2);

% Interpolate to find where the incoming
% hvacSetting lies in the noise table.
hvacDbspl = interp1(tableSetting, tableNoise, hvacSettingRTC);

== matlab function Audiopilot_3_5/NoiseEstimationVariant/SpeedOnly/LfNoiseEstimator/SpeedBoundsAndNoiseSlew/LfNoiseSlew/Decay/sec2sample ==
  data: u input; y output; DecRate parameter
  events: trigger input FUNCTION_CALL_EVENT
function y = fcn(u, DecRate)
% Convert rate from per second to per sample

y = -abs(u.Value/DecRate);

== matlab function Audiopilot_3_5/NoiseEstimationVariant/SpeedOnly/LfNoiseEstimator/SpeedBoundsAndNoiseSlew/LfNoiseSlew/SlowSlew/sec2sample ==
  data: u input; y output; DecRate parameter
  events: trigger input FUNCTION_CALL_EVENT
function y = fcn(u, DecRate)
% Convert rate from per sec to per sample

y = u.Value/DecRate;

== matlab function Audiopilot_3_5/ConfigurationRtcInputs/Hvac/table/TableFormatting ==
  data: tableTOP output; table input; MaskHvacTableSize parameter
  events: trigger input FUNCTION_CALL_EVENT
function tableTOP  = fcn(table, MaskHvacTableSize)
    %#codegen

    % "table": Table containing noise values corresponding to different HVAC
    % settings. Column 1 contains the 'HVAC Setting' and varies from
    % [0,1.0]. Column 2 contains the corresponding 'HVAC noise' values.
    % Error checks for the HVAC table:
    % 1. Column1 must have atleast 2 unique values.
    % 2. Each unique value in column 1 can correspond to only one noise value.
    %    Example- An HVAC setting of 0.5 cannot correspond to both 60 dBSPL and 70 dBSPL.
    % 3. If there are duplicate pairs in the table, only one is retained.
    % 4. Column2 values are expected to either increase with an increase in HVAC setting or remain constant.
    %    Example - The noise corresponding to an HVAC setting of 1.0 must be 
    %    higher than or equal to that of 0.5.
    % 5. If the table does not contain the entries for HVAC settings 0.0 or
    %    1.0, they are added in the translation so that the interpolation
    %    can handle any incoming control messages in the range [0.0, 1.0].
    %    Example - [0.5,70 ; 
    % 6. Size restrictions - the table must have 2 columns and <= MaskHvacTableSize rows.    
    
    % "tableTOP": Output table [16x2] after performing checks

    argName = 'AudioPilot 3.5 HVAC';
    tableTOP = zeros(MaskHvacTableSize,2,'single');
    numEntries = table.Size(1);
    table = table.Value(1:numEntries,:);

    % Sort the table with respect to the fan setting (ascending). 
    % Ensure that the corresponding noise values are also in the ascending 
    % order by checking if the difference between consecutive elements is 
    % always non negative.
    table = sortrows(table,1);
    isNoiseIncreasing = all(diff(table(:,2)) >= 0);
    if ~isNoiseIncreasing
        TranslateError('Error in %s: Noise values must increase with increase in fan current.',argName);
    end
    
    % Ensure that the lowest fan setting is 0 and the highest is 1.0 for
    % the interpolation to work. Using an intermediate variable to add the
    % new row.
    if table(1,1) ~= single(0.0)
        numRows = size(table,1) + 1;
        updatedTable = zeros(numRows,2,'single');
        updatedTable(1,1) = 0.0;
        updatedTable(1,2) = table(1,2);
        updatedTable(2:numRows,:) = table;
        table = updatedTable;
    end
    if table(end,1) ~= single(1.0)
        numRows = size(table,1) + 1;
        updatedTable = zeros(numRows,2,'single');
        updatedTable(numRows,1) = 1.0;
        updatedTable(numRows,2) = table(numRows-1,2);
        updatedTable(1:numRows-1,:) = table;
        table = updatedTable;
    end
    fanSetting = table(:,1);
    noise = table(:,2);
    numEntries = numel(fanSetting);
    
    % Check for unique indexes in fan settings. If a fan setting has a
    % duplicate, check if the corresponding noise values are the same. If
    % they are the same, then only one pair is retained and the others
    % discarded. If they are different, an error is thrown as one fan
    % setting cannot correspond to multiple noise values.
    [fanSettingUnique,idxUnique] = unique(fanSetting);
    duplicateIdx = setdiff(1:numEntries,idxUnique);
    
    for i = 1:numel(duplicateIdx)
        currFanSetting = fanSetting(duplicateIdx(i));
        dupNoise = noise( fanSetting == currFanSetting );
        IsCorrespondingNoiseEqual = all(dupNoise == dupNoise(1));
        if IsCorrespondingNoiseEqual ~= 1
            TranslateError('Error in %s: Fan settings [%f] corresponds to multiple noise values. Ensure that each fan setting corresponds only to one noise value.',argName,currFanSetting);
        end
    end 
    
    numEntriesUnique = numel(fanSettingUnique);
    noiseUnique = noise(idxUnique);
    
    % Number of table entries needs to be atleast 2 for the interp1 function to
    % work and less than equal to MaskHvacTableSize. The fan setting can
    % only be in the range [0,1.0].
    if (numEntriesUnique < 2)
        TranslateError('Error in %s: Noise table must have atleast 2 unique fan settings.',argName);
    end
    if (numEntriesUnique > MaskHvacTableSize)
        TranslateError('Error in %s: Noise table cannot be longer than [%d].', argName,MaskHvacTableSize);
    end
    if (any(fanSetting > 1) || any(fanSetting < 0))
        TranslateError('Error in %s: Fan setting needs to be between 0 and 1.', argName);
    end
    
    % Create the output TOP matrix 
    tableTOP(1:numEntriesUnique,1) = fanSettingUnique;
    tableTOP(1:numEntriesUnique,2) = noiseUnique;
    
end
